simulink model "test_single_pll"  (R2018b)
settings: Solver=FixedStepAuto  StartTime=0.0  StopTime=1  FixedStep=ts  RelTol=1e-3
InitFcn:
  | ts = 1e-3;
undefined symbols (not defined in the file): DiscIntNeverNeededParam
settings Model: Creator=dengzhe  LastModifiedBy=dengzhe

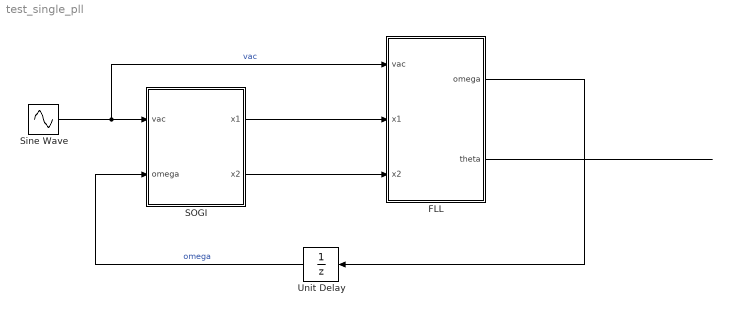
== system test_single_pll ==
  FLL : Subsystem  mask{gamma=0}
  SOGI : Subsystem  mask{k1=1}
  Sine Wave : Sin  Amplitude=220*sqrt(2)  Frequency=2*pi*50  SampleTime=0
  Unit Delay : UnitDelay  SampleTime=-1
  wires:
  Sine Wave/1 -> FLL/1(vac), SOGI/1(vac)  "vac"
  FLL/1(omega) -> Unit Delay/1
  SOGI/1(x1) -> FLL/2(x1)
  SOGI/2(x2) -> FLL/3(x2)
  Unit Delay/1 -> SOGI/2(omega)  "omega"
  FLL/2(theta) -> ?

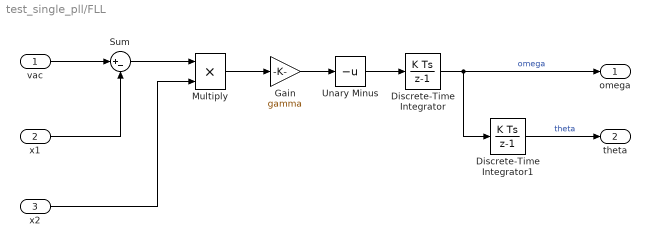
== system test_single_pll/FLL ==
  vac : Inport
  x1 : Inport  Port=2
  x2 : Inport  Port=3
  Discrete-Time Integrator : DiscreteIntegrator  InitialCondition=2*pi*50  SampleTime=ts  ICPrevOutput=DiscIntNeverNeededParam  ICPrevScaledInput=DiscIntNeverNeededParam
  Discrete-Time Integrator1 : DiscreteIntegrator  SampleTime=ts  ICPrevOutput=DiscIntNeverNeededParam  ICPrevScaledInput=DiscIntNeverNeededParam
  Gain : Gain  Gain=gamma
  Multiply : Product
  Sum : Sum  Inputs=|+-
  Unary Minus : UnaryMinus
  omega : Outport
  theta : Outport  Port=2
  wires:
  vac/1 -> Sum/1
  x1/1 -> Sum/2
  Sum/1 -> Multiply/1
  x2/1 -> Multiply/2
  Multiply/1 -> Gain/1
  Gain/1 -> Unary Minus/1
  Discrete-Time Integrator/1 -> Discrete-Time Integrator1/1, omega/1  "omega"
  Unary Minus/1 -> Discrete-Time Integrator/1
  Discrete-Time Integrator1/1 -> theta/1  "theta"

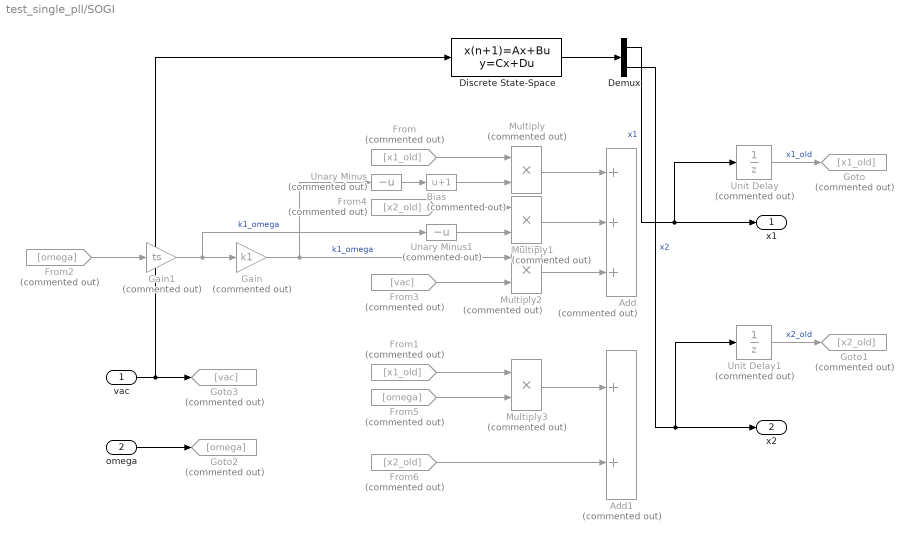
== system test_single_pll/SOGI ==
  vac : Inport
  omega : Inport  Port=2
  Add : Sum  Commented=on  Inputs=3
  Add1 : Sum  Commented=on  Inputs=2
  Bias : Bias  Commented=on  Bias=1
  Demux : Demux  Outputs=2
  Discrete State-Space : DiscreteStateSpace  A=[0.6924, -0.265842; 0.265842, 0.958242]  B=[265.842; 41.7583]  C=[0.0008462, -0.000132921; 0.000132921, 0.000979121]  D=[0.132921; 0.0208791]  SampleTime=-1
  From : From  Commented=on  GotoTag=x1_old
  From1 : From  Commented=on  GotoTag=x1_old
  From2 : From  Commented=on  GotoTag=omega
  From3 : From  Commented=on  GotoTag=vac
  From4 : From  Commented=on  GotoTag=x2_old
  From5 : From  Commented=on  GotoTag=omega
  From6 : From  Commented=on  GotoTag=x2_old
  Gain : Gain  Commented=on  Gain=k1
  Gain1 : Gain  Commented=on  Gain=ts
  Goto : Goto  Commented=on  GotoTag=x1_old
  Goto1 : Goto  Commented=on  GotoTag=x2_old
  Goto2 : Goto  Commented=on  GotoTag=omega
  Goto3 : Goto  Commented=on  GotoTag=vac
  Multiply{,1..3} (4 alike) : Product  Commented=on
  Unary Minus : UnaryMinus  Commented=on
  Unary Minus1 : UnaryMinus  Commented=on
  Unit Delay : UnitDelay  Commented=on  SampleTime=ts
  Unit Delay1 : UnitDelay  Commented=on  SampleTime=ts
  x1 : Outport
  x2 : Outport  Port=2
  wires:
  Unary Minus/1 -> Bias/1
  From/1 -> Multiply/1
  Unit Delay1/1 -> Goto1/1  "x2_old"
  From2/1 -> Gain1/1
  From6/1 -> Add1/2
  Demux/2 -> x2/1, Unit Delay1/1  "x2"
  From4/1 -> Multiply1/1
  omega/1 -> Goto2/1
  vac/1 -> Goto3/1, Discrete State-Space/1
  Gain/1 -> Multiply2/1, Unary Minus/1  "k1_omega"
  From1/1 -> Multiply3/1
  From3/1 -> Multiply2/2
  Bias/1 -> Multiply/2
  Demux/1 -> x1/1, Unit Delay/1  "x1"
  From5/1 -> Multiply3/2
  Multiply2/1 -> Add/3
  Multiply3/1 -> Add1/1
  Multiply/1 -> Add/1
  Unit Delay/1 -> Goto/1  "x1_old"
  Multiply1/1 -> Add/2
  Unary Minus1/1 -> Multiply1/2
  Gain1/1 -> Unary Minus1/1, Gain/1  "k1_omega"
  Discrete State-Space/1 -> Demux/1
